simulink model "es_scheduler_Stateflow"  (R2021a)
settings: Solver=FixedStepDiscrete  StartTime=0.0  StopTime=10.0  FixedStep=10^-3  RelTol=1e-3
libraries: simulink x2
settings Model: Creator=User_LABORATORIO  LastModifiedBy=User_LABORATORIO

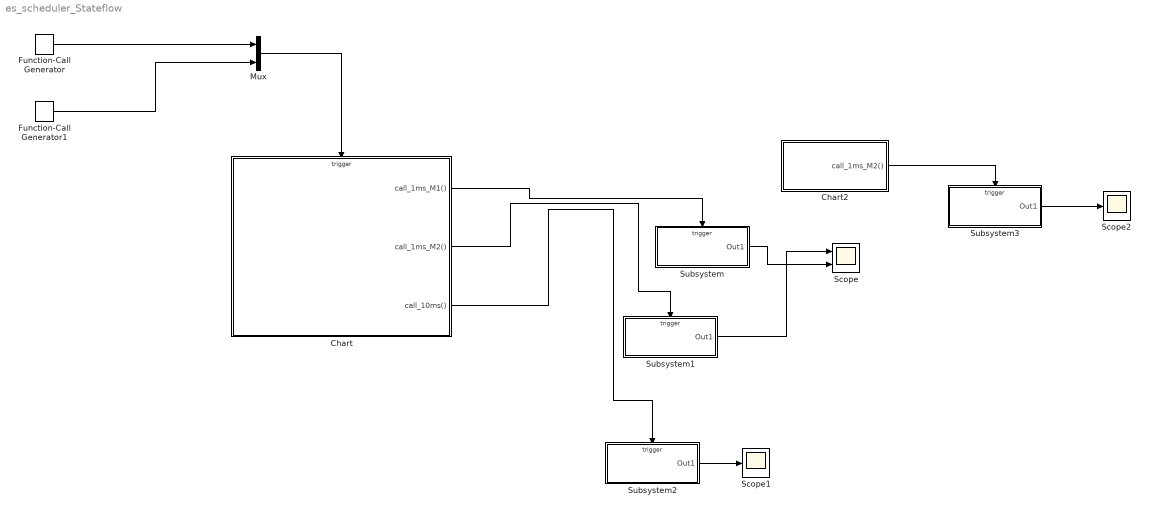
== system es_scheduler_Stateflow ==
  Chart : Stateflow chart  TreatAsAtomicUnit=on
  Chart2 : Stateflow chart  TreatAsAtomicUnit=on
  Function-Call Generator : simulink/Ports & Subsystems/Function-Call Generator  sample_time=0.001  numberOfIterations=1  DisallowWideOutput=off
  Function-Call Generator1 : simulink/Ports & Subsystems/Function-Call Generator  sample_time=0.01  numberOfIterations=1  DisallowWideOutput=off
  Mux : Mux  Inputs=2
  Scope : Scope  NumInputPorts=2
  Scope1 : Scope
  Scope2 : Scope
  Subsystem : Subsystem
  Subsystem1 : Subsystem
  Subsystem2 : Subsystem
  Subsystem3 : Subsystem
  wires:
  Subsystem/1(Out1) -> Scope/2
  Subsystem1/1(Out1) -> Scope/1
  Subsystem2/1(Out1) -> Scope1/1
  Chart2/1(call_1ms_M2()) -> Subsystem3/Trigger
  Subsystem3/1(Out1) -> Scope2/1
  Mux/1 -> Chart/Trigger
  Function-Call Generator/1 -> Mux/1
  Function-Call Generator1/1 -> Mux/2
  Chart/1(call_1ms_M1()) -> Subsystem/Trigger
  Chart/2(call_1ms_M2()) -> Subsystem1/Trigger
  Chart/3(call_10ms()) -> Subsystem2/Trigger

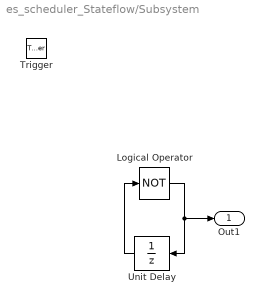
== system es_scheduler_Stateflow/Subsystem ==
  Trigger : TriggerPort  TriggerType=function-call  VariantControl=(inherit)  PortDimensions=1
  Logical Operator : Logic  Operator=NOT  AllPortsSameDT=off  OutDataTypeStr=boolean
  Unit Delay : UnitDelay  SampleTime=-1  HasFrameUpgradeWarning=on
  Out1 : Outport
  wires:
  Logical Operator/1 -> Out1/1, Unit Delay/1
  Unit Delay/1 -> Logical Operator/1

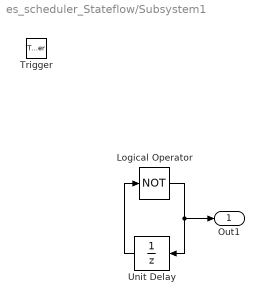
== system es_scheduler_Stateflow/Subsystem1 ==
  Trigger : TriggerPort  TriggerType=function-call  VariantControl=(inherit)  PortDimensions=1
  Logical Operator : Logic  Operator=NOT  AllPortsSameDT=off  OutDataTypeStr=boolean
  Unit Delay : UnitDelay  SampleTime=-1  HasFrameUpgradeWarning=on
  Out1 : Outport
  wires:
  Unit Delay/1 -> Logical Operator/1
  Logical Operator/1 -> Unit Delay/1, Out1/1

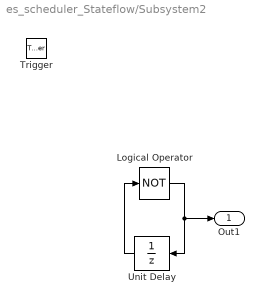
== system es_scheduler_Stateflow/Subsystem2 ==
  Trigger : TriggerPort  TriggerType=function-call  VariantControl=(inherit)  PortDimensions=1
  Logical Operator : Logic  Operator=NOT  AllPortsSameDT=off  OutDataTypeStr=boolean
  Unit Delay : UnitDelay  SampleTime=-1  HasFrameUpgradeWarning=on
  Out1 : Outport
  wires:
  Logical Operator/1 -> Out1/1, Unit Delay/1
  Unit Delay/1 -> Logical Operator/1

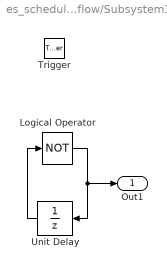
== system es_scheduler_Stateflow/Subsystem3 ==
  Trigger : TriggerPort  TriggerType=function-call  VariantControl=(inherit)  PortDimensions=1
  Logical Operator : Logic  Operator=NOT  AllPortsSameDT=off  OutDataTypeStr=boolean
  Unit Delay : UnitDelay  SampleTime=-1  HasFrameUpgradeWarning=on
  Out1 : Outport
  wires:
  Unit Delay/1 -> Logical Operator/1
  Logical Operator/1 -> Unit Delay/1, Out1/1

== stateflow chart es_scheduler_Stateflow/Chart2 ==
  (default) -> (junction 1)
  (junction 1) -> (junction 3) : {call_1ms_M2;}
  events: call_1ms_M2 output FUNCTION_CALL_EVENT

== stateflow chart es_scheduler_Stateflow/Chart ==
  (default) -> (junction 9)
  (junction 9) -> (junction 11) [order 1] : ev_1ms
  (junction 9) -> (junction 13) [order 2]
  (junction 11) -> (junction 16) : {call_1ms_M1;
      | call_1ms_M2;}
  (junction 13) -> (junction 16) : ev_10ms
      | {call_10ms;}
  (junction 16) -> (junction 21)
  events: ev_1ms input FUNCTION_CALL_EVENT; ev_10ms input FUNCTION_CALL_EVENT; call_1ms_M1 output FUNCTION_CALL_EVENT; call_1ms_M2 output FUNCTION_CALL_EVENT; call_10ms output FUNCTION_CALL_EVENT
